simulink model "ADAC_AEBS_FailOperationTest_A1_cs"  (R2014b)
settings: Solver=ode5  SolverMode=SingleTasking  StartTime=0.0  StopTime=inf  FixedStep=1/100  RelTol=1e-3
PreLoadFcn:
  | mbxruntime.callbacks.PreLoadFcn(bdroot);
  | check_NUTS_defined;
  | 
  | assignin('base',['model_closed_' bdroot],false);addpath('../includes_AEBS');
PostLoadFcn:
  | mbxruntime.callbacks.PostLoadFcn(bdroot);
InitFcn:
  | mbxruntime.callbacks.InitFcn(bdroot);
StartFcn:
  | mbxruntime.callbacks.StartFcn(bdroot);
StopFcn:
  | mbxruntime.callbacks.StopFcn(bdroot);
model workspace: external: MAT-File .\ADAC_AEBS_FailOperationTest_A1_cs_hws.mat (data not in the file)
undefined symbols (not defined in the file or in its folder): OrientationPitch, OrientationRoll, PositionX, PositionY, PositionZ, warningInitialVelocity, x0
undefined symbols (not defined in the file): ADAC_AEBS_FailOperationTest_A1_cs_00c01c95c4c4c5a8, ADAC_AEBS_FailOperationTest_A1_cs_02ad9a283ca297a4, ADAC_AEBS_FailOperationTest_A1_cs_038958de2c1d3e36, ADAC_AEBS_FailOperationTest_A1_cs_05e2aac87d6ae3fd, ADAC_AEBS_FailOperationTest_A1_cs_151e1cb4e3496d77, ADAC_AEBS_FailOperationTest_A1_cs_1ffc4240051d74a2, ADAC_AEBS_FailOperationTest_A1_cs_213e12646a1653ca, ADAC_AEBS_FailOperationTest_A1_cs_235e3212804808b9, ADAC_AEBS_FailOperationTest_A1_cs_2659df7dab90d6e8, ADAC_AEBS_FailOperationTest_A1_cs_2a148b858a6629f8, ADAC_AEBS_FailOperationTest_A1_cs_2b7a9babb669f242, ADAC_AEBS_FailOperationTest_A1_cs_2ed2d4d62929a6bd, ADAC_AEBS_FailOperationTest_A1_cs_33eeee2572576a41, ADAC_AEBS_FailOperationTest_A1_cs_36558e38242c7756, ADAC_AEBS_FailOperationTest_A1_cs_3aef8eead6a1f410, ADAC_AEBS_FailOperationTest_A1_cs_480be3815f0a06c3, ADAC_AEBS_FailOperationTest_A1_cs_4aae23e8cf2dbcb0, ADAC_AEBS_FailOperationTest_A1_cs_5581f50e95ba789b, ADAC_AEBS_FailOperationTest_A1_cs_588f1ee0c5853221, ADAC_AEBS_FailOperationTest_A1_cs_5e60ee4fb7197da0, ADAC_AEBS_FailOperationTest_A1_cs_65b6bc7801839d6b, ADAC_AEBS_FailOperationTest_A1_cs_69e6565dfa73d5e1, ADAC_AEBS_FailOperationTest_A1_cs_745679a1a153644b, ADAC_AEBS_FailOperationTest_A1_cs_78e5010894080216, ADAC_AEBS_FailOperationTest_A1_cs_845ce2ad6322fa97, ADAC_AEBS_FailOperationTest_A1_cs_84cbf4c51e5b1038, ADAC_AEBS_FailOperationTest_A1_cs_884f65c11dfd5d0e, ADAC_AEBS_FailOperationTest_A1_cs_8cda9b0fbfc4f13a, ADAC_AEBS_FailOperationTest_A1_cs_8f45652244c35cb0, ADAC_AEBS_FailOperationTest_A1_cs_8f90241bc576781a, ADAC_AEBS_FailOperationTest_A1_cs_9004477474de018f, ADAC_AEBS_FailOperationTest_A1_cs_9da1e61af7c7ed45, ADAC_AEBS_FailOperationTest_A1_cs_9f73a381d41cec16, ADAC_AEBS_FailOperationTest_A1_cs_a4377d525f2b2f78, ADAC_AEBS_FailOperationTest_A1_cs_ac08e6a613097827, ADAC_AEBS_FailOperationTest_A1_cs_b06a0c6552896264, ADAC_AEBS_FailOperationTest_A1_cs_b268ff1743ece6da, ADAC_AEBS_FailOperationTest_A1_cs_b9108cb16aee3d64, ADAC_AEBS_FailOperationTest_A1_cs_b98118e3e5f7f1f2, ADAC_AEBS_FailOperationTest_A1_cs_BMW_X5_1_Path_pathUniqueID, ADAC_AEBS_FailOperationTest_A1_cs_c19d74ba2d8ab478, ADAC_AEBS_FailOperationTest_A1_cs_c5dbf489b6bc4bea, ADAC_AEBS_FailOperationTest_A1_cs_cde4e91f980952bb, ADAC_AEBS_FailOperationTest_A1_cs_cfc610e8a2cbc10e, ADAC_AEBS_FailOperationTest_A1_cs_e1b1ef473e3d1633, ADAC_AEBS_FailOperationTest_A1_cs_e22c635f60181eec, ADAC_AEBS_FailOperationTest_A1_cs_ea153c165ad4000b, ADAC_AEBS_FailOperationTest_A1_cs_f56ce50e9b4a8f60, ADAC_AEBS_FailOperationTest_A1_cs_f962feabd0e92d60, ADAC_AEBS_FailOperationTest_A1_cs_fea1f748316d75b2, ADAC_AEBS_FailOperationTest_A1_cs_ff71773334c394e4, SteeringColumn, SteeringWheel, WheelL0, WheelL1, WheelR0, WheelR1
libraries: simulink x21, simulink_extras x20, PreScanSimulinkLibrary x17, PreScanUsefulBlocks x2
(part 2 of 11)

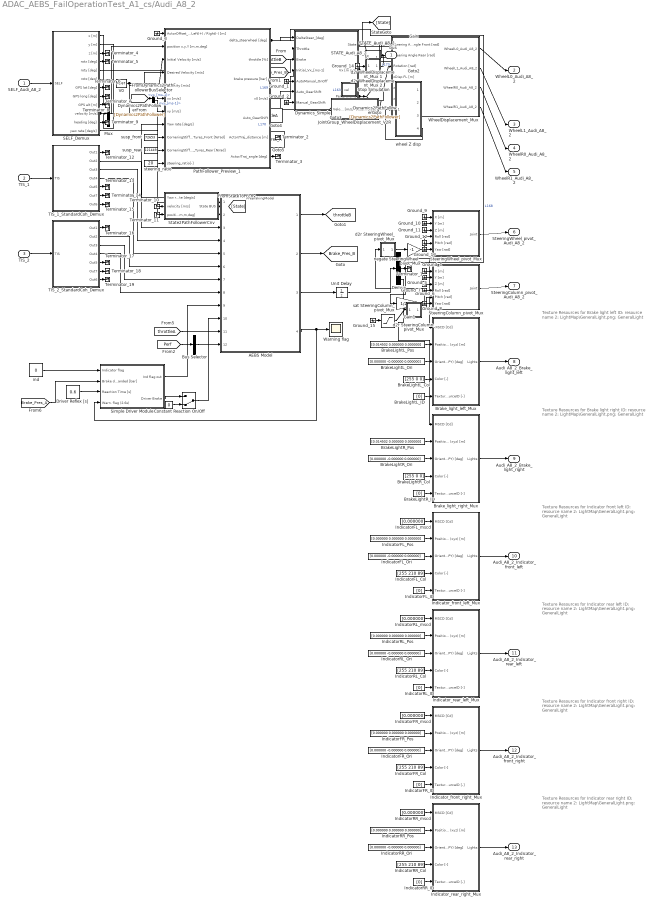
== system ADAC_AEBS_FailOperationTest_A1_cs/Audi_A8_2 ==
  note: Texture Resources for Brake light left
      |
      | ID: resource name
      | 2: LightMap\GeneralLight.png: GeneralLight
  note: Texture Resources for Brake light right
      |
      | ID: resource name
      | 2: LightMap\GeneralLight.png: GeneralLight
  note: Texture Resources for Indicator front left
      |
      | ID: resource name
      | 2: LightMap\GeneralLight.png: GeneralLight
  note: Texture Resources for Indicator rear left
      |
      | ID: resource name
      | 2: LightMap\GeneralLight.png: GeneralLight
  note: Texture Resources for Indicator front right
      |
      | ID: resource name
      | 2: LightMap\GeneralLight.png: GeneralLight
  note: Texture Resources for Indicator rear right
      |
      | ID: resource name
      | 2: LightMap\GeneralLight.png: GeneralLight
  SELF_Audi_A8_2 : Inport  Tag=inport/SelfPort  OutDataTypeStr=Bus: PRESCAN_SELFSENSORDATA  PortDimensions=1  SampleTime=1/100  BusOutputAsStruct=on
  TIS_1 : Inport  Tag=inport/TIS  Port=2  OutDataTypeStr=Bus: PRESCAN_SCANNERSENSOR_MESSAGE  PortDimensions=32  SampleTime=1/25  BusOutputAsStruct=on
  TIS_2 : Inport  Tag=inport/TIS  Port=3  OutDataTypeStr=Bus: PRESCAN_SCANNERSENSOR_MESSAGE  PortDimensions=32  SampleTime=1/25  BusOutputAsStruct=on
  AEBS Model : ModelReference  ModelNameDialog=PreBrakingModel  SimulationMode=Normal  ModelReferenceVersion=1.741  CopyOfModelName=PreBrakingModel  DefaultDataLogging=off
  BrakeLightL_Col : Constant  Tag=VisuLightConst  Value=[255 0 0]
  BrakeLightL_ID : Constant  Tag=VisuLightConst  Value=[0]
  BrakeLightL_Ori : Constant  Tag=VisuLightConst  Value=[0.000000 -0.000000 0.000000]
  BrakeLightL_Pos : Constant  Tag=VisuLightConst  Value=[0.014502 0.000000 0.000000]
  BrakeLightR_Col : Constant  Tag=VisuLightConst  Value=[255 0 0]
  BrakeLightR_ID : Constant  Tag=VisuLightConst  Value=[0]
  BrakeLightR_Ori : Constant  Tag=VisuLightConst  Value=[0.000000 -0.000000 0.000000]
  BrakeLightR_Pos : Constant  Tag=VisuLightConst  Value=[0.014502 0.000000 0.000000]
  Brake_light_left_Mux : Subsystem  Tag=mux/ActiveLight  mask(PreScan User Interface: VisuActiveLight){}
      mask help:
      | The VisuActiveLight block provides a way for detailed animation of Light Sources, such as the indicator, brake, fog and main lights of a vehicle, or a light post.
      |
      | For more information, please click Help.
      settings: DeleteFcn=PreScanBlockDeleteFcn;
      mask Help: eval('openHelp(209)')
  Brake_light_right_Mux : Subsystem  Tag=mux/ActiveLight  mask(PreScan User Interface: VisuActiveLight){}
      mask help:
      | The VisuActiveLight block provides a way for detailed animation of Light Sources, such as the indicator, brake, fog and main lights of a vehicle, or a light post.
      |
      | For more information, please click Help.
      settings: DeleteFcn=PreScanBlockDeleteFcn;
      mask Help: eval('openHelp(209)')
  Bus Selector : BusSelector  OutputSignals=NEngine_[rpm]
  Constant : Constant  Value=0
  Demux : Demux  Outputs=3
  Driver Reflex [s] : Constant  Value=0.6
  Dynamics_Simple : Subsystem  Tag=Simple_Vehicle_Dynamics  mask(PreScan Block: Simple Dynamics){TimeStep=1/100, ComputationMode=Continuous_Time, initialX=ADAC_AEBS_FailOperationTest_A1_cs_4aae23e8cf2dbcb0, initialY=ADAC_AEBS_FailOperationTest_A1_cs_8f90241bc576781a, initialZ=ADAC_AEBS_FailOperationTest_A1_cs_884f65c11dfd5d0e, initialRoll=ADAC_AEBS_FailOperationTest_A1_cs_ff71773334c394e4, initialPitch=ADAC_AEBS_FailOperationTest_A1_cs_05e2aac87d6ae3fd, initialYaw=ADAC_AEBS_FailOperationTest_A1_cs_33eeee2572576a41}
      mask prompts: TimeStep "Auto assigned: Time Step [s]"; ComputationMode "Computation mode:"; initialX "Ini x-position VEHICLE wrt GLOBAL axis system [m]"; initialY "Ini y-position VEHICLE wrt GLOBAL axis system [m]"; initialZ "Ini z-position VEHICLE wrt GLOBAL axis system [m]"; initialRoll "Ini roll-angle BODY wrt VEHICLE axis system [deg]"; initialPitch "Ini pitch-angle BODY wrt VEHICLE axis system [deg]"; initialYaw "Ini yaw-angle VEHICLE wrt GLOBAL axis system [deg]"
      mask help:
      | The Simple Dynamics Model is selected in the GUI to simulate vehicle dynamics behavior.
      |
      | The Simple Dynamics Model is completely open to the user. The parameters of this model can be set in the Simple Dynamics dialog in the GUI.
      |
      | For more information, please click Help.
      mask init:
      | p = SimpleDyn_pars;
      settings: DeleteFcn=PreScanBlockDeleteFcn;
      mask Help: eval('openHelp(220)')
      mask Display:
      | image(imread('SimpleDyn.png'))
      | port_label('input', 1, '{\delta}_S_t_ _e_e_r [deg]','texmode','on')
      | port_label('input', 2, 'Throttle [%]')
      | port_label('input', 3, 'Brake Pres [bar]')
      | port_label('input', 4, 'V_0 [ms-1]','texmode','on')
      | port_label('input', 5, 'Auto=[0]/Manual=[1]')
      | port_label('input', 6, 'Auto_GearShift')
      | port_label('input', 7, 'Manual_GearShift')
      | port_label('output', 1, 'State')
      | port_label('output', 2, 'Vx [ms-1]')
      | port_label('output', 3, 'Perf Params')
  FromDynamics2PathFollowerBusSelector : BusSelector  OutputSignals=vx_[ms-1],vy_[ms-1]
  Gain : Gain  Gain=1/20
  Gain1 : Gain  Gain=1/20
  Ground_{1..15} (15 alike) : Ground
  IndicatorFL_Col : Constant  Tag=VisuLightConst  Value=[255 210 89]
  IndicatorFL_ID : Constant  Tag=VisuLightConst  Value=[0]
  IndicatorFL_Ori : Constant  Tag=VisuLightConst  Value=[0.000000 -0.000000 0.000000]
  IndicatorFL_Pos : Constant  Tag=VisuLightConst  Value=[0.000000 0.000000 0.000000]
  IndicatorFL_mscd : Constant  Tag=VisuLightConst  Value=[0.000000]
  IndicatorFR_Col : Constant  Tag=VisuLightConst  Value=[255 210 89]
  IndicatorFR_ID : Constant  Tag=VisuLightConst  Value=[0]
  IndicatorFR_Ori : Constant  Tag=VisuLightConst  Value=[0.000000 -0.000000 0.000000]
  IndicatorFR_Pos : Constant  Tag=VisuLightConst  Value=[0.000000 0.000000 0.000000]
  IndicatorFR_mscd : Constant  Tag=VisuLightConst  Value=[0.000000]
  IndicatorRL_Col : Constant  Tag=VisuLightConst  Value=[255 210 89]
  IndicatorRL_ID : Constant  Tag=VisuLightConst  Value=[0]
  IndicatorRL_Ori : Constant  Tag=VisuLightConst  Value=[0.000000 -0.000000 0.000000]
  IndicatorRL_Pos : Constant  Tag=VisuLightConst  Value=[0.000000 0.000000 0.000000]
  IndicatorRL_mscd : Constant  Tag=VisuLightConst  Value=[0.000000]
  IndicatorRR_Col : Constant  Tag=VisuLightConst  Value=[255 210 89]
  IndicatorRR_ID : Constant  Tag=VisuLightConst  Value=[0]
  IndicatorRR_Ori : Constant  Tag=VisuLightConst  Value=[0.000000 -0.000000 0.000000]
  IndicatorRR_Pos : Constant  Tag=VisuLightConst  Value=[0.000000 0.000000 0.000000]
  IndicatorRR_mscd : Constant  Tag=VisuLightConst  Value=[0.000000]
  Indicator_front_left_Mux : Subsystem  Tag=mux/ActiveLight  mask(PreScan User Interface: VisuActiveLight){}
      mask help:
      | The VisuActiveLight block provides a way for detailed animation of Light Sources, such as the indicator, brake, fog and main lights of a vehicle, or a light post.
      |
      | For more information, please click Help.
      settings: DeleteFcn=PreScanBlockDeleteFcn;
      mask Help: eval('openHelp(209)')
  Indicator_front_right_Mux : Subsystem  Tag=mux/ActiveLight  mask(PreScan User Interface: VisuActiveLight){}
      mask help:
      | The VisuActiveLight block provides a way for detailed animation of Light Sources, such as the indicator, brake, fog and main lights of a vehicle, or a light post.
      |
      | For more information, please click Help.
      settings: DeleteFcn=PreScanBlockDeleteFcn;
      mask Help: eval('openHelp(209)')
  Indicator_rear_left_Mux : Subsystem  Tag=mux/ActiveLight  mask(PreScan User Interface: VisuActiveLight){}
      mask help:
      | The VisuActiveLight block provides a way for detailed animation of Light Sources, such as the indicator, brake, fog and main lights of a vehicle, or a light post.
      |
      | For more information, please click Help.
      settings: DeleteFcn=PreScanBlockDeleteFcn;
      mask Help: eval('openHelp(209)')
  Indicator_rear_right_Mux : Subsystem  Tag=mux/ActiveLight  mask(PreScan User Interface: VisuActiveLight){}
      mask help:
      | The VisuActiveLight block provides a way for detailed animation of Light Sources, such as the indicator, brake, fog and main lights of a vehicle, or a light post.
      |
      | For more information, please click Help.
      settings: DeleteFcn=PreScanBlockDeleteFcn;
      mask Help: eval('openHelp(209)')
  JointGroup_WheelDisplacement_V2R : Subsystem  Tag=mux/Wheels  mask(PreScan Velocity to Wheel Angle Block:){TimeStep=1/100, TireRadius=0.34}
      mask prompts: TimeStep "Auto Assigned: Time Step [s]"; TireRadius "Tire Radius [m]"
      settings: DeleteFcn=PreScanBlockDeleteFcn;
      mask Display: disp('Velocity\nto\nWheelAngle')
  Mux : Mux  Inputs=3
  PathFollower_Preview_1 : Subsystem  Tag=PathFollower_Preview  mask(PreScan Block: Path Follower with Preview){LongCtrl_P=20, LongCtrl_I=0.3, LongCtrl_D=3.065, LongCtrl_AWU=1, LongCtrlDefault_P=20, LongCtrlDefault_I=0.3, LongCtrlDefault_D=3.065, LongCtrlDefault_AWU=1, PathUniqueID=ADAC_AEBS_FailOperationTest_A1_cs_02ad9a283ca297a4, mass=1820, Jzz=3746, length_a=1.1809, length_l=2.9509, Angle_Max_SteeringWheel=500, PreviewTime=1, DelayTime=0.1, LowSpeedLimit=20, MaxSteeringRate=1200, CSSampleTime=1/100, PFIntegrationFrequency=100}
      mask prompts: LongCtrl_P "Longitudinal Controller P"; LongCtrl_I "Longitudinal Controller I"; LongCtrl_D "Longitudinal Controller D"; LongCtrl_AWU "Longitudinal Controller AWU"; PathUniqueID "Path Unique ID"; mass "Mass vehicle total [kg]"; Jzz "Inertia vehicle around yaw axis [kg m2]"; length_a "Distance between COG and front axle [m]"; length_l "Length of wheelbase [m]"; Angle_Max_SteeringWheel "Maximum steering wheel angle [deg]"; PreviewTime "Preview time [s]"; DelayTime "Delay time [s]"; LowSpeedLimit "Low-speed limit [km/h]"; MaxSteeringRate "Maximum steering wheel angle rate [deg/s]"; CSSampleTime "Compilation Sheet sample time [s]"; PFIntegrationFrequency "Lateral controller frequency [Hz]"
      mask help:
      | The Path Follower Model is selected in the GUI to simulate driver behavior.
      |
      | For more information, please click Help.
      mask init:
      | RefreshCounter = max(floor((1/CSSampleTime) / (PFIntegrationFrequency)), 1);
      | PathFollowerBlockPath = gcb;
      mask Help: eval('openHelp(233)')
      mask DialogControl Control2 Prompt: Reset PID parameters
      mask DialogControl Control2 Callback:
      | LongCtrlDefault_P = get_param(gcb,'LongCtrlDefault_P');
      | set_param(gcb,'LongCtrl_P',LongCtrlDefault_P);
      | 
      | LongCtrlDefault_I = get_param(gcb,'LongCtrlDefault_I');
      | set_param(gcb,'LongCtrl_I',LongCtrlDefault_I);
      | 
      | LongCtrlDefault_D = get_param(gcb,'LongCtrlDefault_D');
      | set_param(gcb,'LongCtrl_D',LongCtrlDefault_D);
      | 
      | LongCtrlDefault_AWU = get_param(gcb,'LongCtrlDefault_AWU');
      | set_param(gcb,'LongCtrl_AWU',LongCtrlDefault_AWU);
  Reaction On/Off : ManualSwitch  CurrentSetting=0
  SELF_Demux : Subsystem  Tag=demux/SelfPort  mask(PreScan Demux Block:){}
      mask help:
      | The SELF port shows (state) information of the actor itself. The outputs are position in the experiment's axis system and the GPS coordinates, and the object's absolute velocity and compass heading.
      |
      | For more information, please click Help.
      settings: DeleteFcn=PreScanBlockDeleteFcn;
      mask Help: eval('openHelp(462)')
      mask Display:
      | port_label('output',1,'x [m]')
      | port_label('output',2,'y [m]')
      | port_label('output',3,'z [m]','texmode','on')
      | port_label('output',4,'Rotx [deg]','texmode','on')
      | port_label('output',5,'Roty [deg]','texmode','on')
      | port_label('output',6,'Rotz [deg]','texmode','on')
      | port_label('output',7,'GPS lat [deg]','texmode','on')
      | port_label('output',8,'GPS long [deg]','texmode','on')
      | port_label('output',9,'GPS alt [m]','texmode','on')
      | port_label('output',10,'Velocity [m/s]')
      | port_label('output',11,'Heading [deg]')
      | port_label('output',12,'Yaw rate [deg/s]')
  STATE_Audi_A8_2_rc : RateTransition  Tag=mux_rc/StatePort  OutPortSampleTimeOpt=Inherit
  Simple Driver Module : Subsystem
  State2PathFollowerCnv : Subsystem  Tag=State2PFConnection/cnv
  SteeringColumn_pivot_Mux : Subsystem  Tag=mux/Joint  mask(PreScan Mux Block){DisplayName=SteeringColumn}
      mask prompts: DisplayName "Display Name"
      mask help:
      | This block simulates a generic joint used for generic models. This joint can be enabled/disabled from the GUI.
      |
      | For more information, please click Help.
      settings: DeleteFcn=PreScanBlockDeleteFcn;
      mask Help: eval('openHelp(254)')
  SteeringWheel_pivot_Mux : Subsystem  Tag=mux/Joint  mask(PreScan Mux Block){DisplayName=SteeringWheel}
      mask prompts: DisplayName "Display Name"
      mask help:
      | This block simulates a generic joint used for generic models. This joint can be enabled/disabled from the GUI.
      |
      | For more information, please click Help.
      settings: DeleteFcn=PreScanBlockDeleteFcn;
      mask Help: eval('openHelp(254)')
  Stop Simulation : Subsystem
  TIS_1_StandardCoh_Demux : Subsystem  Tag=demux/TIS/StandardCoh  TreatAsAtomicUnit=on  mask(PreScan Demux Block: TIS){MAXMESSAGES=32}
      mask prompts: MAXMESSAGES "Number of Objects"
      mask Help: eval('openHelp(449)')
      mask Display:
      | port_label('input',1,'TIS')
      | port_label('output',1,'Beam ID [-]')
      | port_label('output',2,'Range [m]')
      | port_label('output',3,'DopplerVelocity [m/s]')
      | port_label('output',4,'{\theta} [deg]','texmode','on')
      | port_label('output',5,'{\phi} [deg]','texmode','on')
      | port_label('output',6,'Target ID [-]','texmode','on')
      | port_label('output',7,'TIS Data','texmode','on')
  TIS_2_StandardCoh_Demux : Subsystem  Tag=demux/TIS/StandardCoh  TreatAsAtomicUnit=on  mask(PreScan Demux Block: TIS){MAXMESSAGES=32}
      mask prompts: MAXMESSAGES "Number of Objects"
      mask Help: eval('openHelp(449)')
      mask Display:
      | port_label('input',1,'TIS')
      | port_label('output',1,'Beam ID [-]')
      | port_label('output',2,'Range [m]')
      | port_label('output',3,'DopplerVelocity [m/s]')
      | port_label('output',4,'{\theta} [deg]','texmode','on')
      | port_label('output',5,'{\phi} [deg]','texmode','on')
      | port_label('output',6,'Target ID [-]','texmode','on')
      | port_label('output',7,'TIS Data','texmode','on')
  Terminator_{1..19} (19 alike) : Terminator
  Unit Delay : UnitDelay  SampleTime=-1
  V0 : Constant  Value=16.67
  Warning flag : Scope
      settings: TimeRange=1.8  YMin=-1  YMax=1
  WheelDisplacement_Mux : Subsystem  Tag=mux/JointGroup  mask(JointGroup){}
      mask help:
      | The JointGroup allows to control several Joints in one go, as defined for this particular model.
      | For more information, look in the PreScan manual in the section "Model Preparation Tool" -> "Joint Groups"
      |
      | For more information on the Joints simulink interface, press Help.
      mask Help: eval('openHelp(254)')
  d2r SteeringColumn_pivot_Mux : Subsystem  mask(DegreesToRadians){}
      mask help: SimulinkBlocks:simulink_extras:DegreesToRadians_MD
      mask Help: web([docroot '/simulink/ref_extras/degreestoradians.html'])
      mask Display: disp('D2R')
  d2r SteeringWheel_pivot_Mux : Subsystem  mask(DegreesToRadians){}
      mask help: SimulinkBlocks:simulink_extras:DegreesToRadians_MD
      mask Help: web([docroot '/simulink/ref_extras/degreestoradians.html'])
      mask Display: disp('D2R')
  d2r WheelDisplacement_Mux 1 : Subsystem  mask(DegreesToRadians){}
      mask help: SimulinkBlocks:simulink_extras:DegreesToRadians_MD
      mask Help: web([docroot '/simulink/ref_extras/degreestoradians.html'])
      mask Display: disp('D2R')
  d2r WheelDisplacement_Mux 2 : Subsystem  mask(DegreesToRadians){}
      mask help: SimulinkBlocks:simulink_extras:DegreesToRadians_MD
      mask Help: web([docroot '/simulink/ref_extras/degreestoradians.html'])
      mask Display: disp('D2R')
  ind : Constant  Value=0
  negate SteeringWheel_pivot_Mux : Gain  Gain=-1
  sat SteeringColumn_pivot_Mux : Saturate  UpperLimit=30  LowerLimit=-5
  steering_ratio : Constant  Tag=steering_ratio  Value=20
  susp_front : Constant  Tag=susp_front  Value=72653
  susp_rear : Constant  Tag=susp_rear  Value=121449
  wheel Z disp : Subsystem  mask{a=1.17, b=1.77}
      mask prompts: a "Distance to the front wheel from cars center of gravity [m]"; b "Distance to the back wheel from cars center of gravity [m]"
      mask help: Simple Dynamics parameters
  STATE_Audi_A8_2_bus : Outport  Tag=outport/StatePort  OutDataTypeStr=Bus: PRESCAN_STATEACTUATORDATA  PortDimensions=1  SampleTime=1/100
  WheelL0_Audi_A8_2 : Outport  Tag=outport/JointActuator  Port=2  OutDataTypeStr=Bus: PRESCAN_POSE_DATA  SampleTime=1/100
  WheelL1_Audi_A8_2 : Outport  Tag=outport/JointActuator  Port=3  OutDataTypeStr=Bus: PRESCAN_POSE_DATA  SampleTime=1/100
  WheelR0_Audi_A8_2 : Outport  Tag=outport/JointActuator  Port=4  OutDataTypeStr=Bus: PRESCAN_POSE_DATA  SampleTime=1/100
  WheelR1_Audi_A8_2 : Outport  Tag=outport/JointActuator  Port=5  OutDataTypeStr=Bus: PRESCAN_POSE_DATA  SampleTime=1/100
  SteeringWheel_pivot_Audi_A8_2 : Outport  Tag=outport/JointActuator  Port=6  OutDataTypeStr=Bus: PRESCAN_POSE_DATA  SampleTime=1/100
  SteeringColumn_pivot_Audi_A8_2 : Outport  Tag=outport/JointActuator  Port=7  OutDataTypeStr=Bus: PRESCAN_POSE_DATA  SampleTime=1/100
  Audi_A8_2_Brake_light_left : Outport  Tag=outport/BrakeLightL  Port=8  OutDataTypeStr=Bus: PRESCAN_VISULIGHTACTUATOR_DATA  SampleTime=1/100
  Audi_A8_2_Brake_light_right : Outport  Tag=outport/BrakeLightR  Port=9  OutDataTypeStr=Bus: PRESCAN_VISULIGHTACTUATOR_DATA  SampleTime=1/100
  Audi_A8_2_Indicator_front_left : Outport  Tag=outport/IndicatorFL  Port=10  OutDataTypeStr=Bus: PRESCAN_VISULIGHTACTUATOR_DATA  SampleTime=1/100
  Audi_A8_2_Indicator_rear_left : Outport  Tag=outport/IndicatorRL  Port=11  OutDataTypeStr=Bus: PRESCAN_VISULIGHTACTUATOR_DATA  SampleTime=1/100
  Audi_A8_2_Indicator_front_right : Outport  Tag=outport/IndicatorFR  Port=12  OutDataTypeStr=Bus: PRESCAN_VISULIGHTACTUATOR_DATA  SampleTime=1/100
  Audi_A8_2_Indicator_rear_right : Outport  Tag=outport/IndicatorRR  Port=13  OutDataTypeStr=Bus: PRESCAN_VISULIGHTACTUATOR_DATA  SampleTime=1/100
  tag scope: Brake_Pres_A=global, Brake_Pres_B=global, Perf=global, throttleA=global, throttleB=global, view=global
  wires:
  AEBS Model/1 -> [throttleB]
  AEBS Model/2 -> [Brake_Pres_B]
  AEBS Model/3 -> Unit Delay/1
  Unit Delay/1 -> Demux/1
  AEBS Model/4 -> Simple Driver Module/4(Warn. flag (2.6s)), Warning flag/1
  Simple Driver Module/1(Ind flag out) -> AEBS Model/9
  Simple Driver Module/2(Driver Brake) -> Reaction On/Off/1
  Reaction On/Off/1 -> AEBS Model/10
  Constant/1 -> Reaction On/Off/2
  ind/1 -> Simple Driver Module/1(Indicator flag)
  [Brake_Pres_A] -> Simple Driver Module/2(Brake demanded [bar])
  Driver Reflex [s]/1 -> Simple Driver Module/3(Reaction Time [s])
  [throttleA] -> AEBS Model/11
  Bus Selector/1 -> AEBS Model/12
  [Perf] -> Bus Selector/1
  Demux/1 -> Brake_light_left_Mux/1(MSCD [Cd])
  Demux/3 -> Brake_light_right_Mux/1(MSCD [Cd])
  SELF_Demux/10(velocity [m/s]) -> AEBS Model/1, PathFollower_Preview_1/5(velocity [m/s])
  SELF_Demux/12(yaw rate [deg/s]) -> AEBS Model/2
  TIS_1_StandardCoh_Demux/2(Out2) -> AEBS Model/3
  TIS_1_StandardCoh_Demux/3(Out3) -> AEBS Model/4
  TIS_1_StandardCoh_Demux/4(Out4) -> AEBS Model/5
  TIS_2_StandardCoh_Demux/2(Out2) -> AEBS Model/6
  TIS_2_StandardCoh_Demux/3(Out3) -> AEBS Model/7
  TIS_2_StandardCoh_Demux/4(Out4) -> AEBS Model/8
  [throttleB] -> Dynamics_Simple/2(Throttle)
  [Brake_Pres_B] -> Dynamics_Simple/3(Brake)
  Gain/1 -> d2r WheelDisplacement_Mux 1/1(Degrees in)
  d2r WheelDisplacement_Mux 1/1(Radians out) -> WheelDisplacement_Mux/1(Steering Angle Front [rad])
  PathFollower_Preview_1/1(delta_steerwheel [deg]) -> Gain/1, Gain1/1, Dynamics_Simple/1(DeltaSteer_[deg])  "L168"
  Gain1/1 -> d2r SteeringWheel_pivot_Mux/1(Degrees in)
  d2r SteeringWheel_pivot_Mux/1(Radians out) -> negate SteeringWheel_pivot_Mux/1
  negate SteeringWheel_pivot_Mux/1 -> SteeringWheel_pivot_Mux/4(Roll [rad])
  Dynamics_Simple/1(State) -> [view], STATE_Audi_A8_2_rc/1, [State]  "L173"
  Dynamics_Simple/3(Perf_Params) -> [Perf], [Dynamics2PathFollower]
  PathFollower_Preview_1/2(throttle [%]) -> [throttleA]  "L169"
  PathFollower_Preview_1/3(brake pressure [bar]) -> [Brake_Pres_A]  "L170"
  Mux/1 -> PathFollower_Preview_1/2(position x,y,Y [m,m,deg])
  SELF_Demux/1(x [m]) -> Mux/1
  SELF_Demux/2(y [m]) -> Mux/2
  SELF_Demux/6(rotz [deg]) -> Mux/3
  Dynamics_Simple/2(Vx [m s-1]) -> Stop Simulation/1(vel), JointGroup_WheelDisplacement_V2R/1(Velocity [m/s])  "L163"
  V0/1 -> PathFollower_Preview_1/3(Initial Velocity [m/s]), PathFollower_Preview_1/4(Desired Velocity [m/s])
  sat SteeringColumn_pivot_Mux/1 -> d2r SteeringColumn_pivot_Mux/1(Degrees in)
  d2r SteeringColumn_pivot_Mux/1(Radians out) -> SteeringColumn_pivot_Mux/5(Pitch [rad])
  d2r WheelDisplacement_Mux 2/1(Radians out) -> WheelDisplacement_Mux/2(Steering Angle Rear [rad])
  wheel Z disp/1(zDisp FL [m]) -> WheelDisplacement_Mux/4(zDisp FL [m])
  wheel Z disp/2(zDisp FR [m]) -> WheelDisplacement_Mux/5(zDisp FR [m])
  wheel Z disp/3(zDisp RL [m]) -> WheelDisplacement_Mux/6(zDisp RL [m])
  wheel Z disp/4(zDisp RR [m]) -> WheelDisplacement_Mux/7(zDisp RR [m])
  SELF_Demux/5(roty [deg]) -> wheel Z disp/1(rotY [deg])
  STATE_Audi_A8_2_rc/1 -> STATE_Audi_A8_2_bus/1
  SELF_Audi_A8_2/1 -> SELF_Demux/1(SELF)
  TIS_1/1 -> TIS_1_StandardCoh_Demux/1(TIS)
  TIS_2/1 -> TIS_2_StandardCoh_Demux/1(TIS)
  WheelDisplacement_Mux/1(WheelL0_Audi_A8_2) -> WheelL0_Audi_A8_2/1
  WheelDisplacement_Mux/2(WheelL1_Audi_A8_2) -> WheelL1_Audi_A8_2/1
  WheelDisplacement_Mux/3(WheelR0_Audi_A8_2) -> WheelR0_Audi_A8_2/1
  WheelDisplacement_Mux/4(WheelR1_Audi_A8_2) -> WheelR1_Audi_A8_2/1
  JointGroup_WheelDisplacement_V2R/1(Rotation [rad]) -> WheelDisplacement_Mux/3(Rotation [rad])
  SteeringWheel_pivot_Mux/1(Joint) -> SteeringWheel_pivot_Audi_A8_2/1
  SteeringColumn_pivot_Mux/1(Joint) -> SteeringColumn_pivot_Audi_A8_2/1
  Brake_light_left_Mux/1(Lights) -> Audi_A8_2_Brake_light_left/1
  BrakeLightL_Pos/1 -> Brake_light_left_Mux/2(Position (xyz) [m])
  BrakeLightL_Ori/1 -> Brake_light_left_Mux/3(Orientation (RPY) [deg])
  BrakeLightL_Col/1 -> Brake_light_left_Mux/4(Color [-])
  BrakeLightL_ID/1 -> Brake_light_left_Mux/5(TextureResourceID [-])
  Brake_light_right_Mux/1(Lights) -> Audi_A8_2_Brake_light_right/1
  BrakeLightR_Pos/1 -> Brake_light_right_Mux/2(Position (xyz) [m])
  BrakeLightR_Ori/1 -> Brake_light_right_Mux/3(Orientation (RPY) [deg])
  BrakeLightR_Col/1 -> Brake_light_right_Mux/4(Color [-])
  BrakeLightR_ID/1 -> Brake_light_right_Mux/5(TextureResourceID [-])
  Indicator_front_left_Mux/1(Lights) -> Audi_A8_2_Indicator_front_left/1
  IndicatorFL_mscd/1 -> Indicator_front_left_Mux/1(MSCD [Cd])
  IndicatorFL_Pos/1 -> Indicator_front_left_Mux/2(Position (xyz) [m])
  IndicatorFL_Ori/1 -> Indicator_front_left_Mux/3(Orientation (RPY) [deg])
  IndicatorFL_Col/1 -> Indicator_front_left_Mux/4(Color [-])
  IndicatorFL_ID/1 -> Indicator_front_left_Mux/5(TextureResourceID [-])
  Indicator_rear_left_Mux/1(Lights) -> Audi_A8_2_Indicator_rear_left/1
  IndicatorRL_mscd/1 -> Indicator_rear_left_Mux/1(MSCD [Cd])
  IndicatorRL_Pos/1 -> Indicator_rear_left_Mux/2(Position (xyz) [m])
  IndicatorRL_Ori/1 -> Indicator_rear_left_Mux/3(Orientation (RPY) [deg])
  IndicatorRL_Col/1 -> Indicator_rear_left_Mux/4(Color [-])
  IndicatorRL_ID/1 -> Indicator_rear_left_Mux/5(TextureResourceID [-])
  Indicator_front_right_Mux/1(Lights) -> Audi_A8_2_Indicator_front_right/1
  IndicatorFR_mscd/1 -> Indicator_front_right_Mux/1(MSCD [Cd])
  IndicatorFR_Pos/1 -> Indicator_front_right_Mux/2(Position (xyz) [m])
  IndicatorFR_Ori/1 -> Indicator_front_right_Mux/3(Orientation (RPY) [deg])
  IndicatorFR_Col/1 -> Indicator_front_right_Mux/4(Color [-])
  IndicatorFR_ID/1 -> Indicator_front_right_Mux/5(TextureResourceID [-])
  Indicator_rear_right_Mux/1(Lights) -> Audi_A8_2_Indicator_rear_right/1
  IndicatorRR_mscd/1 -> Indicator_rear_right_Mux/1(MSCD [Cd])
  IndicatorRR_Pos/1 -> Indicator_rear_right_Mux/2(Position (xyz) [m])
  IndicatorRR_Ori/1 -> Indicator_rear_right_Mux/3(Orientation (RPY) [deg])
  IndicatorRR_Col/1 -> Indicator_rear_right_Mux/4(Color [-])
  IndicatorRR_ID/1 -> Indicator_rear_right_Mux/5(TextureResourceID [-])
  susp_front/1 -> PathFollower_Preview_1/9(CorneringStiffness_Tyres_Front [N/rad])
  susp_rear/1 -> PathFollower_Preview_1/10(CorneringStiffness_Tyres_Rear [N/rad])
  steering_ratio/1 -> PathFollower_Preview_1/11(steering_ratio[-])
  [State] -> State2PathFollowerCnv/1(State BUS)
  State2PathFollowerCnv/1(Yaw rate [deg/s]) -> PathFollower_Preview_1/8(Yaw rate [deg/s])
  PathFollower_Preview_1/4(v0 [m/s]) -> Dynamics_Simple/4(Initial_Vx_[ms-1])
  PathFollower_Preview_1/5(Auto_GearShift) -> Dynamics_Simple/6(Auto_GearShift)
  FromDynamics2PathFollowerBusSelector/1 -> PathFollower_Preview_1/6(vx [m/s])  "<vx_[ms-1]>"
  FromDynamics2PathFollowerBusSelector/2 -> PathFollower_Preview_1/7(vy [m/s])  "<vy_[ms-1]>"
  [Dynamics2PathFollower] -> FromDynamics2PathFollowerBusSelector/1
  Demux/2 -> Terminator_1/1
  Ground_1/1 -> Dynamics_Simple/5(AutoManual_OnOff)
  Ground_2/1 -> Dynamics_Simple/7(Manual_GearShift)
  Ground_3/1 -> PathFollower_Preview_1/1(ActorOffset_Left(+) / Right(-) [m])
  PathFollower_Preview_1/6(Actor/Traj_distance [m]) -> Terminator_2/1
  PathFollower_Preview_1/7(Actor/Traj_angle [deg]) -> Terminator_3/1
  SELF_Demux/3(z [m]) -> Terminator_4/1
  SELF_Demux/4(rotx [deg]) -> Terminator_5/1
  SELF_Demux/7(GPS lat [deg]) -> Terminator_6/1
  SELF_Demux/8(GPS long [deg]) -> Terminator_7/1
  SELF_Demux/9(GPS alt [m]) -> Terminator_8/1
  SELF_Demux/11(heading [deg]) -> Terminator_9/1
  State2PathFollowerCnv/2(velocity [m/s]) -> Terminator_10/1
  State2PathFollowerCnv/3(position x,y,Y [m,m,deg]) -> Terminator_11/1
  Ground_4/1 -> SteeringColumn_pivot_Mux/1(X [m])
  Ground_5/1 -> SteeringColumn_pivot_Mux/2(Y [m])
  Ground_6/1 -> SteeringColumn_pivot_Mux/3(Z [m])
  Ground_7/1 -> SteeringColumn_pivot_Mux/4(Roll [rad])
  Ground_8/1 -> SteeringColumn_pivot_Mux/6(Yaw [rad])
  Ground_9/1 -> SteeringWheel_pivot_Mux/1(X [m])
  Ground_10/1 -> SteeringWheel_pivot_Mux/2(Y [m])
  Ground_11/1 -> SteeringWheel_pivot_Mux/3(Z [m])
  Ground_12/1 -> SteeringWheel_pivot_Mux/5(Pitch [rad])
  Ground_13/1 -> SteeringWheel_pivot_Mux/6(Yaw [rad])
  TIS_1_StandardCoh_Demux/1(Out1) -> Terminator_12/1
  TIS_1_StandardCoh_Demux/5(Out5) -> Terminator_13/1
  TIS_1_StandardCoh_Demux/6(Out7) -> Terminator_14/1
  TIS_1_StandardCoh_Demux/7(Out6) -> Terminator_15/1
  TIS_2_StandardCoh_Demux/1(Out1) -> Terminator_16/1
  TIS_2_StandardCoh_Demux/5(Out5) -> Terminator_17/1
  TIS_2_StandardCoh_Demux/6(Out7) -> Terminator_18/1
  TIS_2_StandardCoh_Demux/7(Out6) -> Terminator_19/1
  Ground_14/1 -> d2r WheelDisplacement_Mux 2/1(Degrees in)
  Ground_15/1 -> sat SteeringColumn_pivot_Mux/1

== system ADAC_AEBS_FailOperationTest_A1_cs/Audi_A8_2_Brake_light_left ==
  Audi_A8_2_Brake_light_left : Inport  Tag=inport/BrakeLightL  OutDataTypeStr=Bus: PRESCAN_VISULIGHTACTUATOR_DATA  SampleTime=1/100  BusOutputAsStruct=on
  Actuator : S-Function  FunctionName=sfun_VisuLightActuator  Parameters=mbxruntime.parameters.convert(UniqueID), mbxruntime.parameters.convert(LightName), mbxruntime.parameters.convert(PivotName), mbxruntime.parameters.convert(TextureResources), mbxruntime.parameters.convert(ColorsObjectName), mbxruntime.parameters.convert(MeshOnColor), mbxruntime.parameters.convert(MeshOffColor),tabledata, TimeStep  EnableBusSupport=off  mask(PreScan Sink Block: VisuActiveLight){UniqueID=73, LightName=Audi_A8_2.LightActuator_0_BrakeLightRL_ActiveLight, PivotName=Audi_A8_2.BrakeLightL_pivot, TextureResources={ '2' 'LightMap\GeneralLight.png'}, ColorsObjectName=Audi_A8_2.BrakeLightRL, MeshOnColor=[255    0    0  255  255    0    0  255  102  102  102  255  510    0    0  255], MeshOffColor=[255    0    0  255  255    0    0  255  102  102  102  255    0    0    0  255], TimeStep=1/100}
      mask prompts: UniqueID "Parent Unique Identifier"; LightName "Light"; PivotName "Pivot"; TextureResources "Texture Resources"; ColorsObjectName "Light Fixture Color Object"; MeshOnColor "Light Fixture On Color"; MeshOffColor "Light Fixture Off Color"; TimeStep "Simulink time step"
      mask help:
      | The VisuActiveLight block provides a way for detailed animation of Light Sources, such as the indicator, brake, fog and main lights of a vehicle, or a light post.
      |
      | For more information, please click Help.
      mask init:
      | [tabledata] = mbxruntime.parameters.table(UniqueID,LightName,PivotName,TextureResources,ColorsObjectName,MeshOnColor,MeshOffColor);
      mask Help: eval('openHelp(209)')
      mask Display: image(imread('HeadLight.png'))
  wires:
  Audi_A8_2_Brake_light_left/1 -> Actuator/1

== system ADAC_AEBS_FailOperationTest_A1_cs/Audi_A8_2_Brake_light_right ==
  Audi_A8_2_Brake_light_right : Inport  Tag=inport/BrakeLightR  OutDataTypeStr=Bus: PRESCAN_VISULIGHTACTUATOR_DATA  SampleTime=1/100  BusOutputAsStruct=on
  Actuator : S-Function  FunctionName=sfun_VisuLightActuator  Parameters=mbxruntime.parameters.convert(UniqueID), mbxruntime.parameters.convert(LightName), mbxruntime.parameters.convert(PivotName), mbxruntime.parameters.convert(TextureResources), mbxruntime.parameters.convert(ColorsObjectName), mbxruntime.parameters.convert(MeshOnColor), mbxruntime.parameters.convert(MeshOffColor),tabledata, TimeStep  EnableBusSupport=off  mask(PreScan Sink Block: VisuActiveLight){UniqueID=73, LightName=Audi_A8_2.LightActuator_1_BrakeLightRR_ActiveLight, PivotName=Audi_A8_2.BrakeLightR_pivot, TextureResources={ '2' 'LightMap\GeneralLight.png'}, ColorsObjectName=Audi_A8_2.BrakeLightRR, MeshOnColor=[255    0    0  255  255    0    0  255  102  102  102  255  510    0    0  255], MeshOffColor=[255    0    0  255  255    0    0  255  102  102  102  255    0    0    0  255], TimeStep=1/100}
      mask prompts: UniqueID "Parent Unique Identifier"; LightName "Light"; PivotName "Pivot"; TextureResources "Texture Resources"; ColorsObjectName "Light Fixture Color Object"; MeshOnColor "Light Fixture On Color"; MeshOffColor "Light Fixture Off Color"; TimeStep "Simulink time step"
      mask help:
      | The VisuActiveLight block provides a way for detailed animation of Light Sources, such as the indicator, brake, fog and main lights of a vehicle, or a light post.
      |
      | For more information, please click Help.
      mask init:
      | [tabledata] = mbxruntime.parameters.table(UniqueID,LightName,PivotName,TextureResources,ColorsObjectName,MeshOnColor,MeshOffColor);
      mask Help: eval('openHelp(209)')
      mask Display: image(imread('HeadLight.png'))
  wires:
  Audi_A8_2_Brake_light_right/1 -> Actuator/1

== system ADAC_AEBS_FailOperationTest_A1_cs/Audi_A8_2_Indicator_front_left ==
  Audi_A8_2_Indicator_front_left : Inport  Tag=inport/IndicatorFL  OutDataTypeStr=Bus: PRESCAN_VISULIGHTACTUATOR_DATA  SampleTime=1/100  BusOutputAsStruct=on
  Actuator : S-Function  FunctionName=sfun_VisuLightActuator  Parameters=mbxruntime.parameters.convert(UniqueID), mbxruntime.parameters.convert(LightName), mbxruntime.parameters.convert(PivotName), mbxruntime.parameters.convert(TextureResources), mbxruntime.parameters.convert(ColorsObjectName), mbxruntime.parameters.convert(MeshOnColor), mbxruntime.parameters.convert(MeshOffColor),tabledata, TimeStep  EnableBusSupport=off  mask(PreScan Sink Block: VisuActiveLight){UniqueID=73, LightName=Audi_A8_2.LightActuator_6_IndicatorFL_ActiveLight, PivotName=Audi_A8_2.IndicatorFL_pivot, TextureResources={ '2' 'LightMap\GeneralLight.png'}, ColorsObjectName=Audi_A8_2.IndicatorFL, MeshOnColor=[255  165    0    0  255  165    0    0  102  102  102  255  510  420  178  255], MeshOffColor=[255  165    0    0  255  165    0    0  102  102  102  255    0    0    0  255], TimeStep=1/100}
      mask prompts: UniqueID "Parent Unique Identifier"; LightName "Light"; PivotName "Pivot"; TextureResources "Texture Resources"; ColorsObjectName "Light Fixture Color Object"; MeshOnColor "Light Fixture On Color"; MeshOffColor "Light Fixture Off Color"; TimeStep "Simulink time step"
      mask help:
      | The VisuActiveLight block provides a way for detailed animation of Light Sources, such as the indicator, brake, fog and main lights of a vehicle, or a light post.
      |
      | For more information, please click Help.
      mask init:
      | [tabledata] = mbxruntime.parameters.table(UniqueID,LightName,PivotName,TextureResources,ColorsObjectName,MeshOnColor,MeshOffColor);
      mask Help: eval('openHelp(209)')
      mask Display: image(imread('HeadLight.png'))
  wires:
  Audi_A8_2_Indicator_front_left/1 -> Actuator/1

== system ADAC_AEBS_FailOperationTest_A1_cs/Audi_A8_2_Indicator_front_right ==
  Audi_A8_2_Indicator_front_right : Inport  Tag=inport/IndicatorFR  OutDataTypeStr=Bus: PRESCAN_VISULIGHTACTUATOR_DATA  SampleTime=1/100  BusOutputAsStruct=on
  Actuator : S-Function  FunctionName=sfun_VisuLightActuator  Parameters=mbxruntime.parameters.convert(UniqueID), mbxruntime.parameters.convert(LightName), mbxruntime.parameters.convert(PivotName), mbxruntime.parameters.convert(TextureResources), mbxruntime.parameters.convert(ColorsObjectName), mbxruntime.parameters.convert(MeshOnColor), mbxruntime.parameters.convert(MeshOffColor),tabledata, TimeStep  EnableBusSupport=off  mask(PreScan Sink Block: VisuActiveLight){UniqueID=73, LightName=Audi_A8_2.LightActuator_8_IndicatorFR_ActiveLight, PivotName=Audi_A8_2.IndicatorFR_pivot, TextureResources={ '2' 'LightMap\GeneralLight.png'}, ColorsObjectName=Audi_A8_2.IndicatorFR, MeshOnColor=[255  165    0    0  255  165    0    0  102  102  102  255  510  420  178  255], MeshOffColor=[255  165    0    0  255  165    0    0  102  102  102  255    0    0    0  255], TimeStep=1/100}
      mask prompts: UniqueID "Parent Unique Identifier"; LightName "Light"; PivotName "Pivot"; TextureResources "Texture Resources"; ColorsObjectName "Light Fixture Color Object"; MeshOnColor "Light Fixture On Color"; MeshOffColor "Light Fixture Off Color"; TimeStep "Simulink time step"
      mask help:
      | The VisuActiveLight block provides a way for detailed animation of Light Sources, such as the indicator, brake, fog and main lights of a vehicle, or a light post.
      |
      | For more information, please click Help.
      mask init:
      | [tabledata] = mbxruntime.parameters.table(UniqueID,LightName,PivotName,TextureResources,ColorsObjectName,MeshOnColor,MeshOffColor);
      mask Help: eval('openHelp(209)')
      mask Display: image(imread('HeadLight.png'))
  wires:
  Audi_A8_2_Indicator_front_right/1 -> Actuator/1

== system ADAC_AEBS_FailOperationTest_A1_cs/Audi_A8_2_Indicator_rear_left ==
  Audi_A8_2_Indicator_rear_left : Inport  Tag=inport/IndicatorRL  OutDataTypeStr=Bus: PRESCAN_VISULIGHTACTUATOR_DATA  SampleTime=1/100  BusOutputAsStruct=on
  Actuator : S-Function  FunctionName=sfun_VisuLightActuator  Parameters=mbxruntime.parameters.convert(UniqueID), mbxruntime.parameters.convert(LightName), mbxruntime.parameters.convert(PivotName), mbxruntime.parameters.convert(TextureResources), mbxruntime.parameters.convert(ColorsObjectName), mbxruntime.parameters.convert(MeshOnColor), mbxruntime.parameters.convert(MeshOffColor),tabledata, TimeStep  EnableBusSupport=off  mask(PreScan Sink Block: VisuActiveLight){UniqueID=73, LightName=Audi_A8_2.LightActuator_7_IndicatorRL_ActiveLight, PivotName=Audi_A8_2.IndicatorRL_pivot, TextureResources={ '2' 'LightMap\GeneralLight.png'}, ColorsObjectName=Audi_A8_2.IndicatorRL, MeshOnColor=[255  165    0    0  255  165    0    0  102  102  102  255  510  420  178  255], MeshOffColor=[255  165    0    0  255  165    0    0  102  102  102  255    0    0    0  255], TimeStep=1/100}
      mask prompts: UniqueID "Parent Unique Identifier"; LightName "Light"; PivotName "Pivot"; TextureResources "Texture Resources"; ColorsObjectName "Light Fixture Color Object"; MeshOnColor "Light Fixture On Color"; MeshOffColor "Light Fixture Off Color"; TimeStep "Simulink time step"
      mask help:
      | The VisuActiveLight block provides a way for detailed animation of Light Sources, such as the indicator, brake, fog and main lights of a vehicle, or a light post.
      |
      | For more information, please click Help.
      mask init:
      | [tabledata] = mbxruntime.parameters.table(UniqueID,LightName,PivotName,TextureResources,ColorsObjectName,MeshOnColor,MeshOffColor);
      mask Help: eval('openHelp(209)')
      mask Display: image(imread('HeadLight.png'))
  wires:
  Audi_A8_2_Indicator_rear_left/1 -> Actuator/1

== system ADAC_AEBS_FailOperationTest_A1_cs/Audi_A8_2_Indicator_rear_right ==
  Audi_A8_2_Indicator_rear_right : Inport  Tag=inport/IndicatorRR  OutDataTypeStr=Bus: PRESCAN_VISULIGHTACTUATOR_DATA  SampleTime=1/100  BusOutputAsStruct=on
  Actuator : S-Function  FunctionName=sfun_VisuLightActuator  Parameters=mbxruntime.parameters.convert(UniqueID), mbxruntime.parameters.convert(LightName), mbxruntime.parameters.convert(PivotName), mbxruntime.parameters.convert(TextureResources), mbxruntime.parameters.convert(ColorsObjectName), mbxruntime.parameters.convert(MeshOnColor), mbxruntime.parameters.convert(MeshOffColor),tabledata, TimeStep  EnableBusSupport=off  mask(PreScan Sink Block: VisuActiveLight){UniqueID=73, LightName=Audi_A8_2.LightActuator_9_IndicatorRR_ActiveLight, PivotName=Audi_A8_2.IndicatorRR_pivot, TextureResources={ '2' 'LightMap\GeneralLight.png'}, ColorsObjectName=Audi_A8_2.IndicatorRR, MeshOnColor=[255  165    0    0  255  165    0    0  102  102  102  255  510  420  178  255], MeshOffColor=[255  165    0    0  255  165    0    0  102  102  102  255    0    0    0  255], TimeStep=1/100}
      mask prompts: UniqueID "Parent Unique Identifier"; LightName "Light"; PivotName "Pivot"; TextureResources "Texture Resources"; ColorsObjectName "Light Fixture Color Object"; MeshOnColor "Light Fixture On Color"; MeshOffColor "Light Fixture Off Color"; TimeStep "Simulink time step"
      mask help:
      | The VisuActiveLight block provides a way for detailed animation of Light Sources, such as the indicator, brake, fog and main lights of a vehicle, or a light post.
      |
      | For more information, please click Help.
      mask init:
      | [tabledata] = mbxruntime.parameters.table(UniqueID,LightName,PivotName,TextureResources,ColorsObjectName,MeshOnColor,MeshOffColor);
      mask Help: eval('openHelp(209)')
      mask Display: image(imread('HeadLight.png'))
  wires:
  Audi_A8_2_Indicator_rear_right/1 -> Actuator/1
